simulink model "MEMS_Gyro_Open_SenseMode"  (R2022b)
settings: Solver=VariableStepAuto  StartTime=0.0  StopTime=10  MaxStep=1e-5  RelTol=1e-3
model workspace (MAT data in the model file):
  Ax = 5e-06
  Kamp = 210
  Kcv = 3.5
  Kyc = 114810
  Qy = 320
  Vr = 1
  a0 = 0
  a1 = -1.57079632679
  my = 6.7e-07
  wd = 24001.7678734
  wy = 24416.4581037
  wyx = 24001.7678734
libraries: dsparch4 x9
settings Model: Creator=Rio  LastModifiedBy=Rio

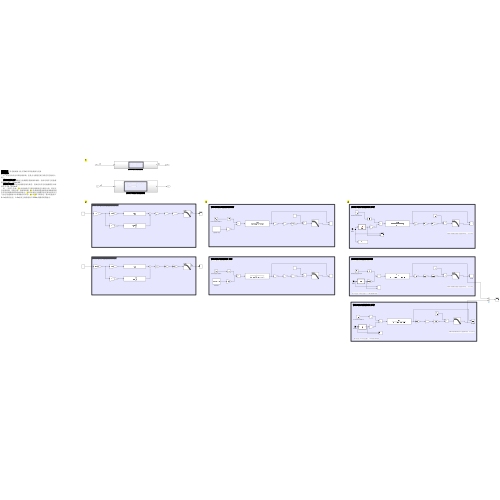
[thumbnail: Simulink's stored preview of the top-level diagram]
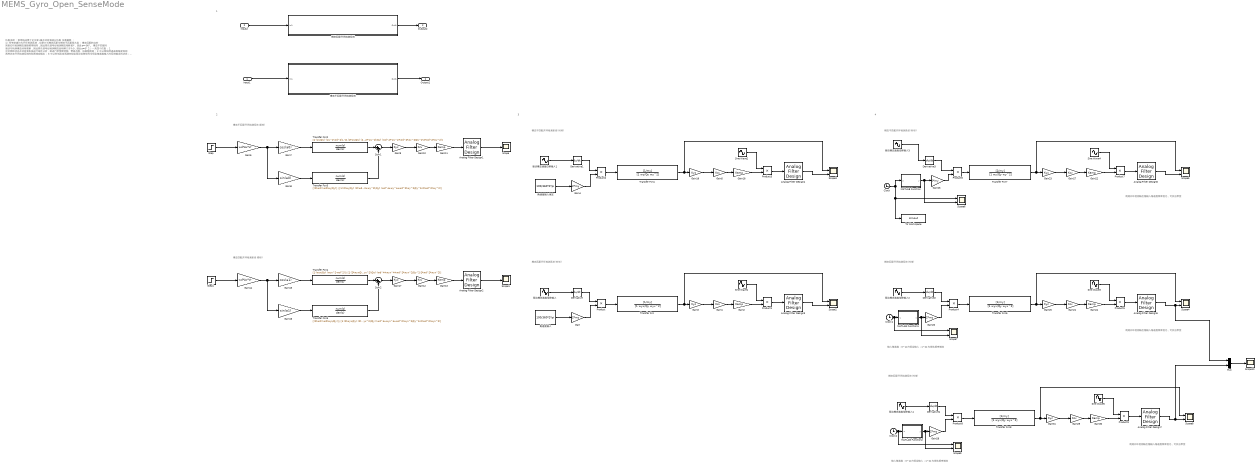
== system MEMS_Gyro_Open_SenseMode ==
  note: 1
  note: 输入角速度：0~1s内恒定输入；1~2s内线性频率增加
  note: 模态匹配开环检测系统(时域)
  note: 仿真说明 ：参考杨成博士论文第4章开环检测部分仿真
      | 仿真解释 ：
      | 1）所有仿真均为开环检测系统，但是分为模态匹配与模态不匹配两大类：
      | 模态匹配特点时 则驱动与检测模态谐振频率相同，因此哥氏信号经检测模态相移90°，因此a=-90°。
      | 模态不匹配时 驱动与检测模态间有频差，因此哥氏信号经检测模态后相移几乎为0，因此a=0°
      | 2）一共四个仿真： 1 中对两种状态开环检测系统进行线性分析，即进行奈奎斯特图、零极点图、伯德图观测； 2 中从频域传递函数角度观测 两种状态开环检测系统的阶跃响应输出； 3 中从时域出发观测在稳定驱动位移信号与恒定角速度输入时系统输出的状态； 4 中较 3 所不同的是，输入角速度在0~1s内保持恒定，1~2s内发生线性增加只150Hz,观测系统的输出。
  note: 模态不匹配开环检测系统(频域)
  note: 模态匹配开环检测系统(频域)
  note: 模态不匹配开环检测系统(时域)
  note: 模态匹配开环检测系统(时域)
  note: 模态不匹配开环检测系统(时域)
  note: 观测开环检测输出随输入角速度频率变化，可反应带宽
  note: 观测开环检测输出随输入角速度频率变化，可反应带宽
  note: 2
  note: 3
  note: 4
  note: 输入角速度：0~1s内恒定输入；1~2s内线性频率增加
  note: 观测开环检测输出随输入角速度频率变化，可反应带宽
  note: 模态匹配开环检测系统(时域)
  Input1 : Inport
  Input2 : Inport  Port=2
  Analog Filter Design1 : dsparch4/Analog Filter Design  method=Butterworth  filttype=Lowpass  N=1  Wlo=2*pi*150  Whi=80  Rp=2  Rs=40
  Analog Filter Design2 : dsparch4/Analog Filter Design  method=Butterworth  filttype=Lowpass  N=1  Wlo=2*pi*150  Whi=80  Rp=2  Rs=40
  Analog Filter Design{3..7} (5 alike) : dsparch4/Analog Filter Design  method=Butterworth  filttype=Lowpass  N=2  Wlo=2*pi*150  Whi=80  Rp=2  Rs=40
  Clock : Clock
  Clock1 : Clock
  Clock2 : Clock
  Derivative{,1..4} (5 alike) : Derivative
  Gain{,4,20,26,28} (5 alike) : Gain  Gain=2*my
  Gain{1,5,10,12,21,27,29} (7 alike) : Gain  Gain=Kcv
  Gain{2,11,13,18,22,24,30} (7 alike) : Gain  Gain=Kamp
  Gain14 : Gain  Gain=wd*Ax*Vr
  Gain15 : Gain  Gain=cos(a1)
  Gain16 : Gain  Gain=sin(a1)
  Gain{3,9,17,19,23,25,31} (7 alike) : Gain  Gain=Kyc
  Gain6 : Gain  Gain=wd*Ax*Vr
  Gain7 : Gain  Gain=cos(a0)
  Gain8 : Gain  Gain=sin(a0)
  MATLAB Function : MATLAB Function  TreatAsAtomicUnit=on
  MATLAB Function1 : MATLAB Function  TreatAsAtomicUnit=on
  MATLAB Function2 : MATLAB Function  TreatAsAtomicUnit=on
  Mux : Mux  Inputs=2
  Product{,1..9} (10 alike) : Product
  Scope : Scope
  Scope1 : Scope
  Scope10 : Scope
  Scope{2..9} (8 alike) : Scope  NumInputPorts=2
  Sine Wave1 : Sin  Frequency=wd  SampleTime=0
  Sine Wave2 : Sin  Frequency=wd  Phase=90  SampleTime=0
  Sine Wave3 : Sin  Frequency=wd  SampleTime=0
  Sine Wave4 : Sin  Frequency=wd  Phase=90  SampleTime=0
  Sine Wave5 : Sin  Frequency=wd  SampleTime=0
  Step : Step  Time=0  SampleTime=0
  Step1 : Step  Time=0  SampleTime=0
  Sum1 : Sum  Inputs=|+-
  Sum2 : Sum  Inputs=|+-
  To Workspace : ToWorkspace  VariableName=simout  SaveFormat=Timeseries  SampleTime=-1
  Transfer Fcn : TransferFcn  Numerator=[1/my]  Denominator=[1 wyx/Qy wyx^2]
  Transfer Fcn1 : TransferFcn  Numerator=[1/my]  Denominator=[1 wy/Qy wy^2]
  Transfer Fcn2 : TransferFcn  Numerator=[1 (wy/Qy) (wy^2-wd^2)]  Denominator=[1 (2*wy/Qy) (2*wd^2+2*wy^2+wy^2/Qy^2) (2*wy*(wd^2+wy^2)/Qy) (wd^4+wy^4+wd^2*wy^2/Qy^2-2*wd^2*wy^2)]
  Transfer Fcn3 : TransferFcn  Numerator=[(2*wd) (wd*wy/Qy)]  Denominator=[1 (2*wy/Qy) (2*wd^2+2*wy^2+wy^2/Qy^2) (2*wy*(wd^2+wy^2)/Qy) (wd^4+wy^4+wd^2*wy^2/Qy^2-2*wd^2*wy^2)]
  Transfer Fcn4 : TransferFcn  Numerator=[1 (wyx/Qy) (wyx^2-wd^2)]  Denominator=[1 (2*wyx/Qy) (2*wd^2+2*wyx^2+wyx^2/Qy^2) (2*wyx*(wd^2+wyx^2)/Qy) (wd^4+wyx^4+wd^2*wyx^2/Qy^2-2*wd^2*wyx^2)]
  Transfer Fcn5 : TransferFcn  Numerator=[(2*wd) (wd*wyx/Qy)]  Denominator=[1 (2*wyx/Qy) (2*wd^2+2*wyx^2+wyx^2/Qy^2) (2*wyx*(wd^2+wyx^2)/Qy) (wd^4+wyx^4+wd^2*wyx^2/Qy^2-2*wd^2*wyx^2)]
  Transfer Fcn6 : TransferFcn  Numerator=[1/my]  Denominator=[1 wyx/Qy wyx^2]
  Transfer Fcn7 : TransferFcn  Numerator=[1/my]  Denominator=[1 wy/Qy wy^2]
  Transfer Fcn8 : TransferFcn  Numerator=[1/my]  Denominator=[1 wyx/Qy wyx^2]
  模态不匹配开环检测系统 : Subsystem
  模态匹配开环检测系统 : Subsystem
  角速度输入 : Constant  Value=100/360*2*pi
  角速度输入恒定 : Constant  Value=100/360*2*pi
  驱动模态速度位移输入{,1..4} (5 alike) : Sin  Amplitude=Ax  Frequency=wd  SampleTime=0
  Output1 : Outport
  Output2 : Outport  Port=2
  wires:
  Analog Filter Design1/1 -> Scope/1
  Gain11/1 -> Analog Filter Design1/1
  Step/1 -> Gain6/1
  Gain6/1 -> Gain8/1, Gain7/1
  Transfer Fcn2/1 -> Sum1/1
  Gain10/1 -> Gain11/1
  Gain8/1 -> Transfer Fcn3/1
  Transfer Fcn3/1 -> Sum1/2
  Gain7/1 -> Transfer Fcn2/1
  Sum1/1 -> Gain9/1
  Gain9/1 -> Gain10/1
  Analog Filter Design2/1 -> Scope1/1
  Step1/1 -> Gain14/1
  Gain13/1 -> Analog Filter Design2/1
  Gain17/1 -> Gain12/1
  Sum2/1 -> Gain17/1
  Gain16/1 -> Transfer Fcn5/1
  Gain15/1 -> Transfer Fcn4/1
  Transfer Fcn5/1 -> Sum2/2
  Transfer Fcn4/1 -> Sum2/1
  Gain14/1 -> Gain16/1, Gain15/1
  Gain12/1 -> Gain13/1
  Input2/1 -> 模态匹配开环检测系统/1(In1)
  模态匹配开环检测系统/1(Out1) -> Output2/1
  Input1/1 -> 模态不匹配开环检测系统/1(In1)
  模态不匹配开环检测系统/1(Out1) -> Output1/1
  驱动模态速度位移输入/1 -> Derivative/1
  角速度输入/1 -> Gain/1
  Derivative/1 -> Product/1
  Gain/1 -> Product/2
  Product/1 -> Transfer Fcn/1
  Transfer Fcn/1 -> Scope2/1, Gain3/1
  Gain3/1 -> Gain1/1
  Gain1/1 -> Gain2/1
  Gain2/1 -> Product1/2
  Sine Wave1/1 -> Product1/1
  Product1/1 -> Analog Filter Design3/1
  Analog Filter Design3/1 -> Scope2/2
  Analog Filter Design4/1 -> Scope3/2
  Transfer Fcn1/1 -> Scope3/1, Gain19/1
  Product3/1 -> Analog Filter Design4/1
  Derivative1/1 -> Product2/1
  Gain5/1 -> Gain18/1
  Gain18/1 -> Product3/2
  Sine Wave2/1 -> Product3/1
  驱动模态速度位移输入1/1 -> Derivative1/1
  角速度输入恒定/1 -> Gain4/1
  Gain4/1 -> Product2/2
  Gain19/1 -> Gain5/1
  Product2/1 -> Transfer Fcn1/1
  Product6/1 -> Transfer Fcn7/1
  Gain23/1 -> Gain27/1
  Gain26/1 -> Product6/2
  驱动模态速度位移输入3/1 -> Derivative3/1
  Sine Wave4/1 -> Product7/1
  Gain22/1 -> Product7/2
  Gain27/1 -> Gain22/1
  Derivative3/1 -> Product6/1
  Product7/1 -> Analog Filter Design6/1
  Transfer Fcn7/1 -> Gain23/1, Scope5/1
  Analog Filter Design6/1 -> Scope5/2
  Analog Filter Design5/1 -> Mux/1, Scope4/2
  Product5/1 -> Analog Filter Design5/1
  Sine Wave3/1 -> Product5/1
  Gain24/1 -> Product5/2
  Gain21/1 -> Gain24/1
  Gain25/1 -> Gain21/1
  Transfer Fcn6/1 -> Gain25/1, Scope4/1
  Product4/1 -> Transfer Fcn6/1
  Gain20/1 -> Product4/2
  Derivative2/1 -> Product4/1
  驱动模态速度位移输入2/1 -> Derivative2/1
  Clock/1 -> Scope6/1, To Workspace/1, MATLAB Function/1(u)
  MATLAB Function/1(y) -> Scope6/2, Gain26/1
  Clock1/1 -> Scope7/1, MATLAB Function1/1(u)
  MATLAB Function1/1(y) -> Scope7/2, Gain20/1
  MATLAB Function2/1(y) -> Scope9/2, Gain28/1
  Clock2/1 -> Scope9/1, MATLAB Function2/1(u)
  Product9/1 -> Analog Filter Design7/1
  驱动模态速度位移输入4/1 -> Derivative4/1
  Derivative4/1 -> Product8/1
  Sine Wave5/1 -> Product9/1
  Product8/1 -> Transfer Fcn8/1
  Gain29/1 -> Gain30/1
  Gain30/1 -> Product9/2
  Analog Filter Design7/1 -> Mux/2, Scope8/2
  Gain31/1 -> Gain29/1
  Gain28/1 -> Product8/2
  Transfer Fcn8/1 -> Gain31/1, Scope8/1
  Mux/1 -> Scope10/1

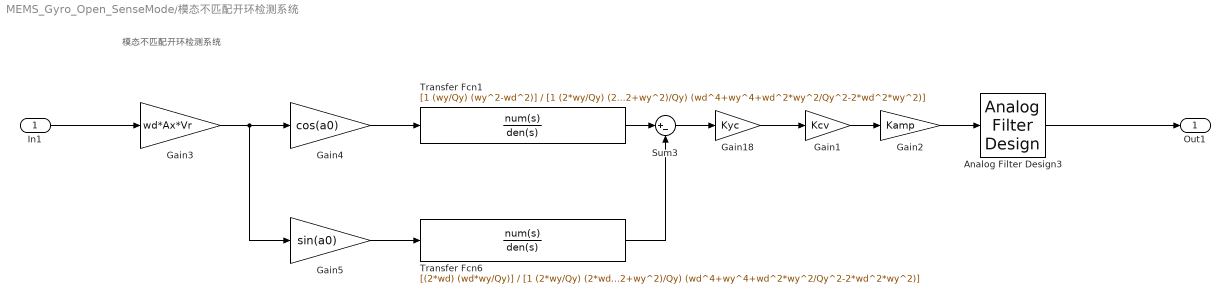
== system MEMS_Gyro_Open_SenseMode/模态不匹配开环检测系统 ==
  note: 模态不匹配开环检测系统
  In1 : Inport
  Analog Filter Design3 : dsparch4/Analog Filter Design  method=Butterworth  filttype=Lowpass  N=1  Wlo=2*pi*150  Whi=80  Rp=2  Rs=40
  Gain1 : Gain  Gain=Kcv
  Gain18 : Gain  Gain=Kyc
  Gain2 : Gain  Gain=Kamp
  Gain3 : Gain  Gain=wd*Ax*Vr
  Gain4 : Gain  Gain=cos(a0)
  Gain5 : Gain  Gain=sin(a0)
  Sum3 : Sum  Inputs=|+-
  Transfer Fcn1 : TransferFcn  Numerator=[1 (wy/Qy) (wy^2-wd^2)]  Denominator=[1 (2*wy/Qy) (2*wd^2+2*wy^2+wy^2/Qy^2) (2*wy*(wd^2+wy^2)/Qy) (wd^4+wy^4+wd^2*wy^2/Qy^2-2*wd^2*wy^2)]
  Transfer Fcn6 : TransferFcn  Numerator=[(2*wd) (wd*wy/Qy)]  Denominator=[1 (2*wy/Qy) (2*wd^2+2*wy^2+wy^2/Qy^2) (2*wy*(wd^2+wy^2)/Qy) (wd^4+wy^4+wd^2*wy^2/Qy^2-2*wd^2*wy^2)]
  Out1 : Outport
  wires:
  Transfer Fcn6/1 -> Sum3/2
  Gain18/1 -> Gain1/1
  Transfer Fcn1/1 -> Sum3/1
  Gain2/1 -> Analog Filter Design3/1
  Sum3/1 -> Gain18/1
  Gain4/1 -> Transfer Fcn1/1
  Gain5/1 -> Transfer Fcn6/1
  Gain3/1 -> Gain5/1, Gain4/1
  Gain1/1 -> Gain2/1
  In1/1 -> Gain3/1
  Analog Filter Design3/1 -> Out1/1

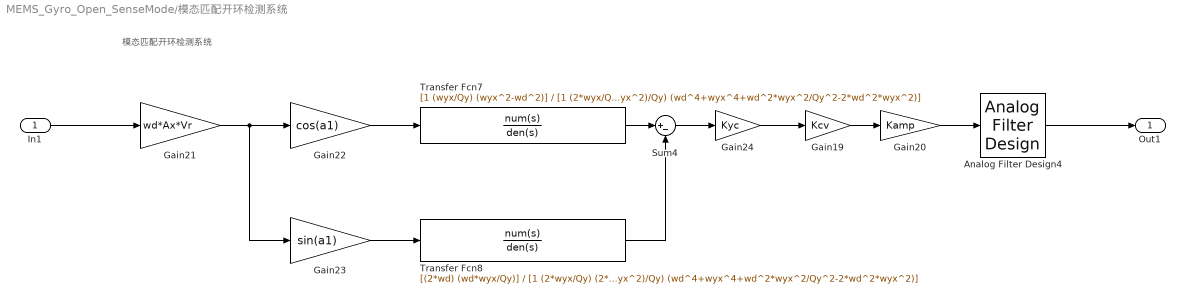
== system MEMS_Gyro_Open_SenseMode/模态匹配开环检测系统 ==
  note: 模态匹配开环检测系统
  In1 : Inport
  Analog Filter Design4 : dsparch4/Analog Filter Design  method=Butterworth  filttype=Lowpass  N=1  Wlo=2*pi*150  Whi=80  Rp=2  Rs=40
  Gain19 : Gain  Gain=Kcv
  Gain20 : Gain  Gain=Kamp
  Gain21 : Gain  Gain=wd*Ax*Vr
  Gain22 : Gain  Gain=cos(a1)
  Gain23 : Gain  Gain=sin(a1)
  Gain24 : Gain  Gain=Kyc
  Sum4 : Sum  Inputs=|+-
  Transfer Fcn7 : TransferFcn  Numerator=[1 (wyx/Qy) (wyx^2-wd^2)]  Denominator=[1 (2*wyx/Qy) (2*wd^2+2*wyx^2+wyx^2/Qy^2) (2*wyx*(wd^2+wyx^2)/Qy) (wd^4+wyx^4+wd^2*wyx^2/Qy^2-2*wd^2*wyx^2)]
  Transfer Fcn8 : TransferFcn  Numerator=[(2*wd) (wd*wyx/Qy)]  Denominator=[1 (2*wyx/Qy) (2*wd^2+2*wyx^2+wyx^2/Qy^2) (2*wyx*(wd^2+wyx^2)/Qy) (wd^4+wyx^4+wd^2*wyx^2/Qy^2-2*wd^2*wyx^2)]
  Out1 : Outport
  wires:
  Gain24/1 -> Gain19/1
  Gain20/1 -> Analog Filter Design4/1
  Gain19/1 -> Gain20/1
  Gain23/1 -> Transfer Fcn8/1
  Gain21/1 -> Gain23/1, Gain22/1
  Transfer Fcn8/1 -> Sum4/2
  Gain22/1 -> Transfer Fcn7/1
  Transfer Fcn7/1 -> Sum4/1
  Sum4/1 -> Gain24/1
  Analog Filter Design4/1 -> Out1/1
  In1/1 -> Gain21/1

== matlab function MEMS_Gyro_Open_SenseMode/MATLAB Function ==
  data: u input; y output
function y = fcn(u)
w=150*2*pi*(u-1);
if(u<1)
    y= 100/360*2*pi;
else
    y = 100/360*2*pi*cos(w*(u-1));
end

== matlab function MEMS_Gyro_Open_SenseMode/MATLAB Function2 ==
  data: u input; y output
function y = fcn(u)
% w=150*2*pi*(u-1);
% if(u<1)
%     y= 100/360*2*pi;
% else
%     y = 100/360*2*pi*cos(w*(u-1));
% end

%%% 变速率
% w=150*2*pi*(u);
% 
% y = 100/360*2*pi*cos(w*(u));

%%% 恒定速率
w=0*2*pi;

y = 100/360*2*pi*cos(w*(u));

== matlab function MEMS_Gyro_Open_SenseMode/MATLAB Function1 ==
  data: u input; y output
function y = fcn(u)
% w=150*2*pi*(u-1);
% if(u<1)
%     y= 100/360*2*pi;
% else
%     y = 100/360*2*pi*cos(w*(u-1));
% end

%%% 变速率
% w=150*2*pi*(u);
% 
% y = 100/360*2*pi*cos(w*(u));

%%% 恒定速率
w=6*2*pi;

y = 100/360*2*pi*cos(w*(u));
